simulink model "ch7example2"  (Simulink 5.0)
settings: Solver=FixedStepDiscrete  StartTime=0.0  StopTime=10.0  FixedStep=1/10  RelTol=1e-3
libraries: commrandsrc2 x1, simulink x1, commutil2 x1
settings Model: LastModifiedBy=shaoyubin

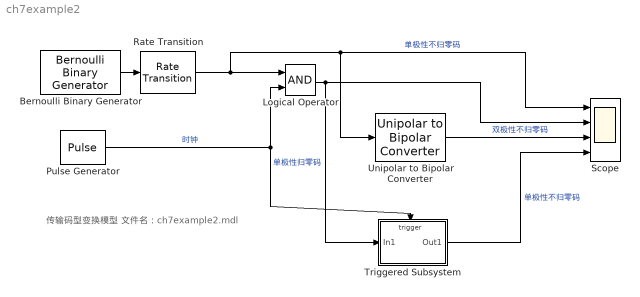
== system ch7example2 ==
  note: 传输码型变换模型
      | 文件名：ch7example2.mdl
  Bernoulli Binary Generator : commrandsrc2/Bernoulli Binary Generator  P=0.5  seed=61  Ts=1  frameBased=off  sampPerFrame=1  orient=off
  Logical Operator : Logic  AllPortsSameDT=off
  Pulse Generator : DiscretePulseGenerator  Period=10  PulseWidth=4  SampleTime=1/10
  Rate Transition : simulink/Signal Attributes/Rate Transition  DataIntegrity=on  DeterministicTransfer=on  TransitionType=Slow to fast  InitCond=0
  Scope : Scope  NumInputPorts=4
      settings: YMin=-2~-2~-2~-2  YMax=2~2~2~2
  Triggered Subsystem : Subsystem  TreatAsAtomicUnit=on
  Unipolar to Bipolar Converter : commutil2/Unipolar to Bipolar Converter  M=2  polarity=Positive
  wires:
  Bernoulli Binary Generator/1 -> Rate Transition/1
  Pulse Generator/1 -> Logical Operator/2, Triggered Subsystem/Trigger  "时钟"
  Rate Transition/1 -> Logical Operator/1, Scope/1, Unipolar to Bipolar Converter/1  "单极性不归零码"
  Unipolar to Bipolar Converter/1 -> Scope/3  "双极性不归零码"
  Logical Operator/1 -> Scope/2, Triggered Subsystem/1(In1)  "单极性归零码"
  Triggered Subsystem/1(Out1) -> Scope/4  "单极性不归零码"

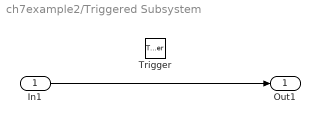
== system ch7example2/Triggered Subsystem ==
  In1 : Inport
  Trigger : TriggerPort
  Out1 : Outport
  wires:
  In1/1 -> Out1/1
